simulink model "posModel1"  (R2021b)
settings: Solver=ode5  StartTime=0.0  StopTime=runT  FixedStep=dt  RelTol=1e-3
InitFcn:
  | posInit1;
values from neighbouring files (symbols this model uses):
  Bm = bm * gearRatio * gearRatio    (= 2.601)    [posInit1.m]    (also in posInit2.m; posInit3.m)
  den1d = cell2mat(posModelDisTF.Denominator)    [posInit1.m]
  den2d = cell2mat(sysEdisTF.Denominator)    [posInit1.m]
  dt = 0.001    [posInit1.m]    (also in posInit2.m; posInit3.m)
  Jm = jm * gearRatio * gearRatio    (= 0.023968215)    [posInit1.m]    (also in posInit2.m; posInit3.m)
  kd = 1    [posInit1.m]    (also in posInit2.m; posInit3.m)
  kp = 50    [posInit1.m]    (also in posInit2.m; posInit3.m = 80)
  num1d = cell2mat(posModelDisTF.Numerator)    [posInit1.m]
  num2d = cell2mat(sysEdisTF.Numerator)    [posInit1.m]
  q0 = 0    [posInit1.m]    (also in posInit2.m; posInit3.m)
  qdot0 = 0    [posInit1.m]    (also in posInit2.m; posInit3.m)
libraries: simulink x2
settings Model: Creator=86135  LastModifiedBy=86135

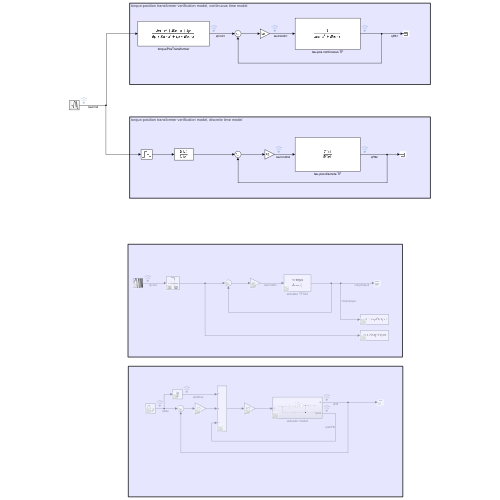
[thumbnail: Simulink's stored preview of the top-level diagram]
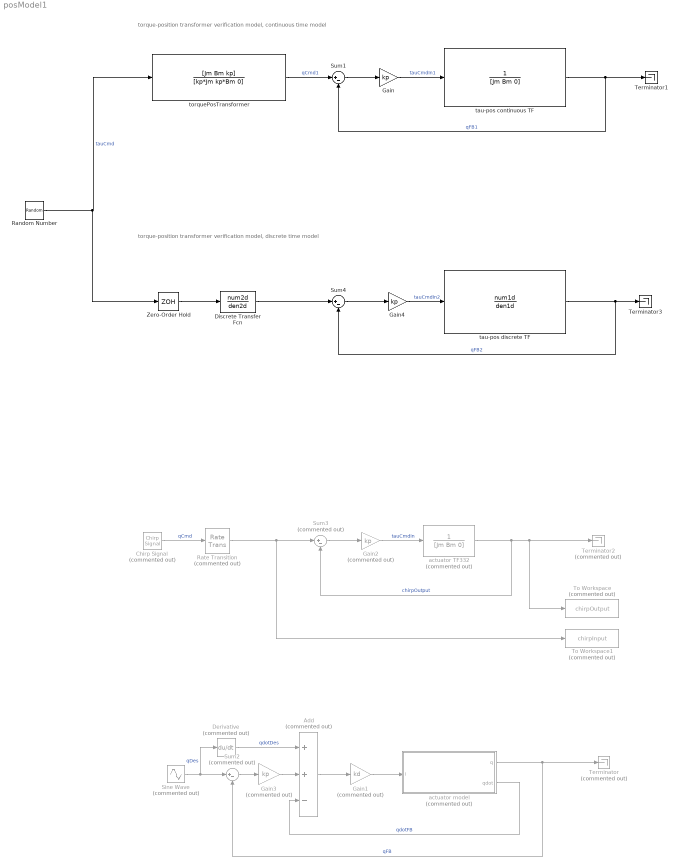
== system posModel1 ==
  note: torque-position transformer verification model, discrete time model
  note: torque-position transformer verification model, continuous time model
  Add : Sum  Commented=on  Inputs=++-
  Chirp Signal : simulink/Sources/Chirp Signal  Commented=on  f1=f0  T=131.071  f2=f1
  Derivative : Derivative  Commented=on
  Discrete Transfer Fcn : DiscreteTransferFcn  Numerator=num2d  Denominator=den2d  SampleTime=dt
  Gain : Gain  Gain=kp
  Gain1 : Gain  Commented=on  Gain=kd
  Gain2 : Gain  Commented=on  Gain=kp
  Gain3 : Gain  Commented=on  Gain=kp
  Gain4 : Gain  Gain=kp
  Random Number : RandomNumber  Variance=5  Seed=16  SampleTime=0.5
  Rate Transition : RateTransition  Commented=on  OutPortSampleTime=0.001
  Sine Wave : Sin  Commented=on  Frequency=2  SampleTime=0
  Sum1 : Sum  Inputs=|+-
  Sum2 : Sum  Commented=on  Inputs=|+-
  Sum3 : Sum  Commented=on  Inputs=|+-
  Sum4 : Sum  Inputs=|+-
  Terminator : Terminator  Commented=on
  Terminator1 : Terminator
  Terminator2 : Terminator  Commented=on
  Terminator3 : Terminator
  To Workspace : ToWorkspace  Commented=on  VariableName=chirpOutput  SaveFormat=Timeseries  SampleTime=-1
  To Workspace1 : ToWorkspace  Commented=on  VariableName=chirpInput  SaveFormat=Timeseries  SampleTime=-1
  Zero-Order Hold : ZeroOrderHold  SampleTime=dt
  actuator TF332 : TransferFcn  Commented=on  Denominator=[Jm Bm 0]
  actuator model : Subsystem  Commented=on
  tau-pos continuous TF : TransferFcn  Denominator=[Jm Bm 0]
  tau-pos discrete TF : DiscreteTransferFcn  Numerator=num1d  Denominator=den1d  SampleTime=dt
  torquePosTransformer : TransferFcn  Numerator=[Jm Bm kp]  Denominator=[kp*Jm kp*Bm 0]
  wires:
  actuator model/1(q) -> Terminator/1, Sum2/2  "qFB"
  Sum2/1 -> Gain3/1
  Sine Wave/1 -> Sum2/1, Derivative/1  "qDes"
  actuator model/2(qdot) -> Add/3  "qdotFB"
  Gain3/1 -> Add/2
  Gain1/1 -> actuator model/1(i)
  Add/1 -> Gain1/1
  Derivative/1 -> Add/1  "qdotDes"
  Gain/1 -> tau-pos continuous TF/1  "tauCmdIn1"
  Sum1/1 -> Gain/1
  tau-pos continuous TF/1 -> Sum1/2, Terminator1/1  "qFB1"
  Random Number/1 -> Zero-Order Hold/1, torquePosTransformer/1  "tauCmd"
  torquePosTransformer/1 -> Sum1/1  "qCmd1"
  Chirp Signal/1 -> Rate Transition/1  "qCmd"
  Sum3/1 -> Gain2/1
  Gain2/1 -> actuator TF332/1  "tauCmdIn"
  Rate Transition/1 -> Sum3/1, To Workspace1/1
  actuator TF332/1 -> Terminator2/1, To Workspace/1, Sum3/2  "chirpOutput"
  Gain4/1 -> tau-pos discrete TF/1  "tauCmdIn2"
  tau-pos discrete TF/1 -> Sum4/2, Terminator3/1  "qFB2"
  Sum4/1 -> Gain4/1
  Discrete Transfer Fcn/1 -> Sum4/1
  Zero-Order Hold/1 -> Discrete Transfer Fcn/1

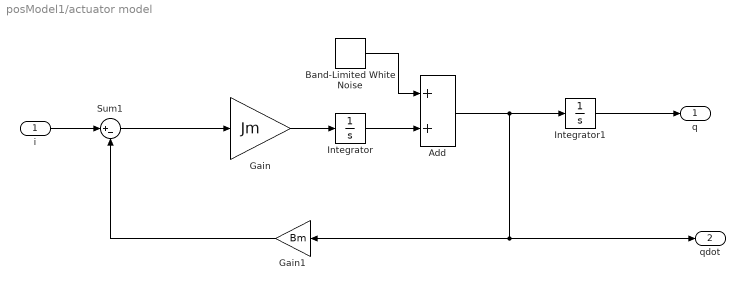
== system posModel1/actuator model ==
  i : Inport
  Add : Sum
  Band-Limited White Noise : simulink/Sources/Band-Limited White Noise  Cov=[0.00001]  Ts=0.001  seed=[16666]
  Gain : Gain  Gain=Jm
  Gain1 : Gain  Gain=Bm
  Integrator : Integrator  InitialCondition=qdot0
  Integrator1 : Integrator  InitialCondition=q0
  Sum1 : Sum  Inputs=|+-
  q : Outport
  qdot : Outport  Port=2
  wires:
  i/1 -> Sum1/1
  Sum1/1 -> Gain/1
  Gain1/1 -> Sum1/2
  Gain/1 -> Integrator/1
  Integrator1/1 -> q/1
  Integrator/1 -> Add/2
  Add/1 -> Gain1/1, qdot/1, Integrator1/1
  Band-Limited White Noise/1 -> Add/1
